simulink model "projekt1_1"  (R2016b)
settings: Solver=VariableStepAuto  StartTime=0.0  StopTime=300.0  RelTol=1e-3
values from neighbouring files (symbols this model uses):
  a1 = 0.56    [projekt1.m]    (also in projekt1_5.m)
  a2 = -0.8    [projekt1.m]    (also in projekt1_5.m)
  a3 = 0.35    [projekt1.m]    (also in projekt1_5.m)
  a4 = 0.2    [projekt1.m]    (also in projekt1_5.m)
  K = 3.5    [projekt1.m]    (also in projekt1_5.m)
  T1 = 4    [projekt1.m]    (also in projekt1_5.m)
  T2 = 8    [projekt1.m]    (also in projekt1_5.m)
settings Model: Creator=m  LastModifiedBy=m

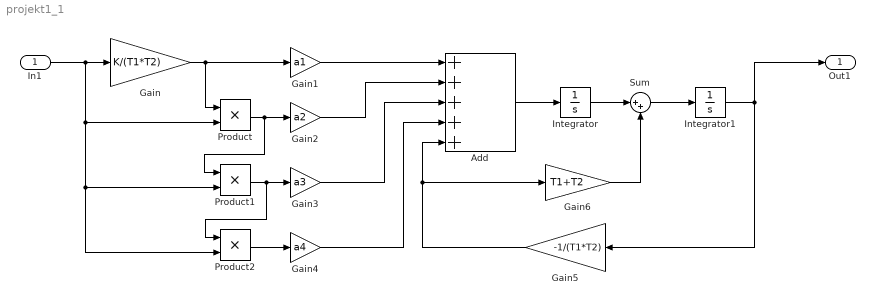
== system projekt1_1 ==
  In1 : Inport
  Add : Sum  Inputs=+++++
  Gain : Gain  Gain=K/(T1*T2)
  Gain1 : Gain  Gain=a1
  Gain2 : Gain  Gain=a2
  Gain3 : Gain  Gain=a3
  Gain4 : Gain  Gain=a4
  Gain5 : Gain  Gain=-1/(T1*T2)
  Gain6 : Gain  Gain=T1+T2
  Integrator : Integrator  ContinuousStateAttributes='x_2'
  Integrator1 : Integrator  ContinuousStateAttributes='x_2'
  Product : Product
  Product1 : Product
  Product2 : Product
  Sum : Sum  Inputs=|++
  Out1 : Outport  SignalName=y(t)
  wires:
  In1/1 -> Product2/2, Product1/2, Product/2, Gain/1
  Gain/1 -> Product/1, Gain1/1
  Product2/1 -> Gain4/1
  Product/1 -> Product1/1, Gain2/1
  Product1/1 -> Product2/1, Gain3/1
  Gain1/1 -> Add/1
  Gain2/1 -> Add/2
  Gain3/1 -> Add/3
  Gain4/1 -> Add/4
  Gain5/1 -> Gain6/1, Add/5
  Add/1 -> Integrator/1
  Integrator/1 -> Sum/1
  Gain6/1 -> Sum/2
  Sum/1 -> Integrator1/1
  Integrator1/1 -> Out1/1, Gain5/1
